simulink model "Linear_Bicycle_Model"  (R2022b)
settings: Solver=ode4  StartTime=0.0  StopTime=20  FixedStep=1e-3  RelTol=1e-3
values from neighbouring files (symbols this model uses):
  Np = 40    [linear_bicycle_script.m]    (also in nonlinear_bicycle_script.m)
  Ts = 0.01    [linear_bicycle_script.m]    (also in nonlinear_bicycle_script.m)
  V_ref = 90 /3.6    (= 25)    [veh_parameters.m]
undefined symbols (not defined in the file or in its folder): data, init, input
settings Model: Creator=nishantc  LastModifiedBy=fiala
settings SolverCC: AlgebraicLoopSolver=TrustRegion
settings DataIOCC: ReturnWorkspaceOutputs=off
settings DebuggingCC: UnconnectedInputMsg=warning  UnconnectedOutputMsg=warning  UnconnectedLineMsg=warning  SFMachineParentedDataDiag=warning  ArithmeticOperatorsInVariantConditions=warning
settings ModelReferenceCC: EnableRefExpFcnMdlSchedulingChecks=on
settings SFSimCC: CustomCodeUndefinedFunction=UseInterfaceOnly
settings RTWCC: DLArmComputeVersion=19.05

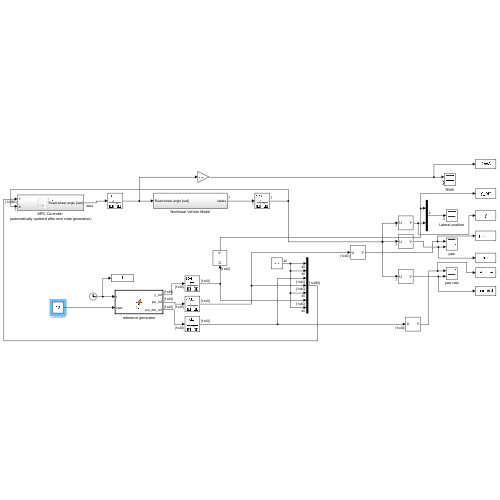
[thumbnail: Simulink's stored preview of the top-level diagram]
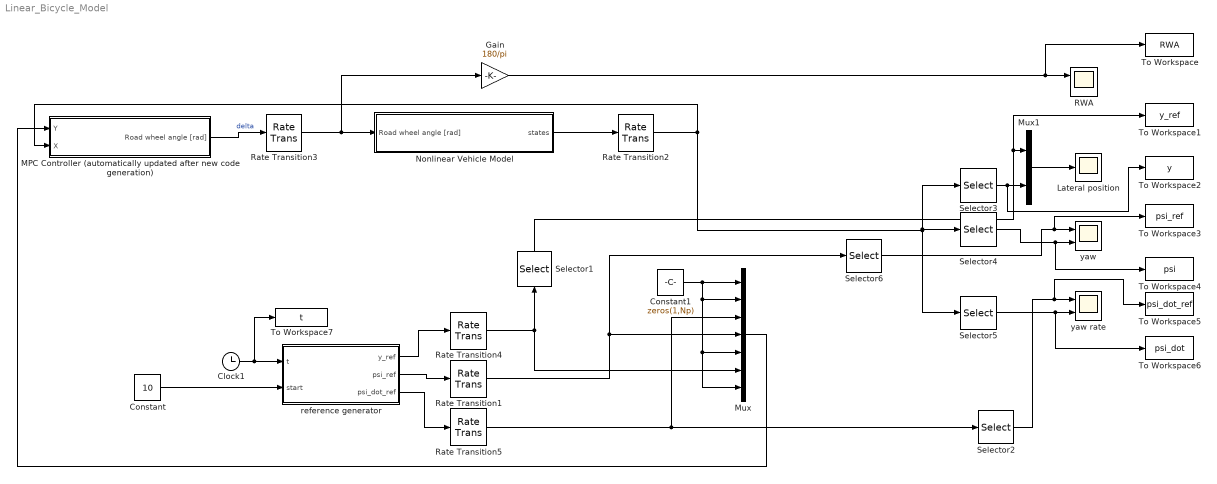
== system Linear_Bicycle_Model ==
  Clock1 : Clock
      settings: Decimation=1000
  Constant : Constant  Value=10
  Constant1 : Constant  Value=zeros(1,Np)
  Gain : Gain  Gain=180/pi
  Lateral position : Scope
  MPC Controller (automatically updated after new code generation) : Subsystem
  Mux : Mux  Inputs=7
  Mux1 : Mux  Inputs=2
  Nonlinear Vehicle Model : Subsystem
  RWA : Scope  NumInputPorts=2
  Rate Transition{1..2,4..5} (4 alike) : RateTransition  OutPortSampleTime=Ts
  Rate Transition3 : RateTransition
  Selector1 : Selector  InputPortWidth=40  IndexOptions=Index vector (dialog)  Indices=1  OutputSizes=1
  Selector2 : Selector  InputPortWidth=40  IndexOptions=Index vector (dialog)  Indices=1  OutputSizes=1
  Selector3 : Selector  InputPortWidth=7  IndexOptions=Index vector (dialog)  Indices=6  OutputSizes=1
  Selector4 : Selector  InputPortWidth=7  IndexOptions=Index vector (dialog)  Indices=4  OutputSizes=1
  Selector5 : Selector  InputPortWidth=7  IndexOptions=Index vector (dialog)  Indices=3  OutputSizes=1
  Selector6 : Selector  InputPortWidth=40  IndexOptions=Index vector (dialog)  Indices=1  OutputSizes=1
  To Workspace : ToWorkspace  VariableName=RWA  SampleTime=-1
  To Workspace1 : ToWorkspace  VariableName=y_ref  SampleTime=-1
  To Workspace2 : ToWorkspace  VariableName=y  SampleTime=-1
  To Workspace3 : ToWorkspace  VariableName=psi_ref  SampleTime=-1
  To Workspace4 : ToWorkspace  VariableName=psi  SampleTime=-1
  To Workspace5 : ToWorkspace  VariableName=psi_dot_ref  SampleTime=-1
  To Workspace6 : ToWorkspace  VariableName=psi_dot  SampleTime=-1
  To Workspace7 : ToWorkspace  VariableName=t  SampleTime=-1
  reference generator : MATLAB Function  TreatAsAtomicUnit=on
  yaw : Scope  NumInputPorts=2
  yaw rate : Scope  NumInputPorts=2
  wires:
  MPC Controller (automatically updated after new code generation)/1(Road wheel angle [rad]) -> Rate Transition3/1  "delta"
  Mux1/1 -> Lateral position/1
  Nonlinear Vehicle Model/1(states) -> Rate Transition2/1
  Selector3/1 -> To Workspace2/1, Mux1/2
  Rate Transition2/1 -> MPC Controller (automatically updated after new code generation)/2(X), Selector3/1, Selector4/1, Selector5/1
  Rate Transition3/1 -> Nonlinear Vehicle Model/1(Road wheel angle [rad]), Gain/1
  Gain/1 -> To Workspace/1, RWA/1
  Mux/1 -> MPC Controller (automatically updated after new code generation)/1(Y)
  Clock1/1 -> To Workspace7/1, reference generator/1(t)
  Constant/1 -> reference generator/2(start)
  reference generator/1(y_ref) -> Rate Transition4/1
  reference generator/2(psi_ref) -> Rate Transition1/1
  reference generator/3(psi_dot_ref) -> Rate Transition5/1
  Selector4/1 -> To Workspace4/1, yaw/2
  Selector5/1 -> To Workspace6/1, yaw rate/2
  Rate Transition1/1 -> Mux/4, Selector6/1
  Rate Transition4/1 -> Selector1/1, Mux/6
  Rate Transition5/1 -> Mux/3, Selector2/1
  Selector1/1 -> To Workspace1/1, Mux1/1
  Selector2/1 -> To Workspace5/1, yaw rate/1
  Selector6/1 -> To Workspace3/1, yaw/1
  Constant1/1 -> Mux/7, Mux/5, Mux/2, Mux/1

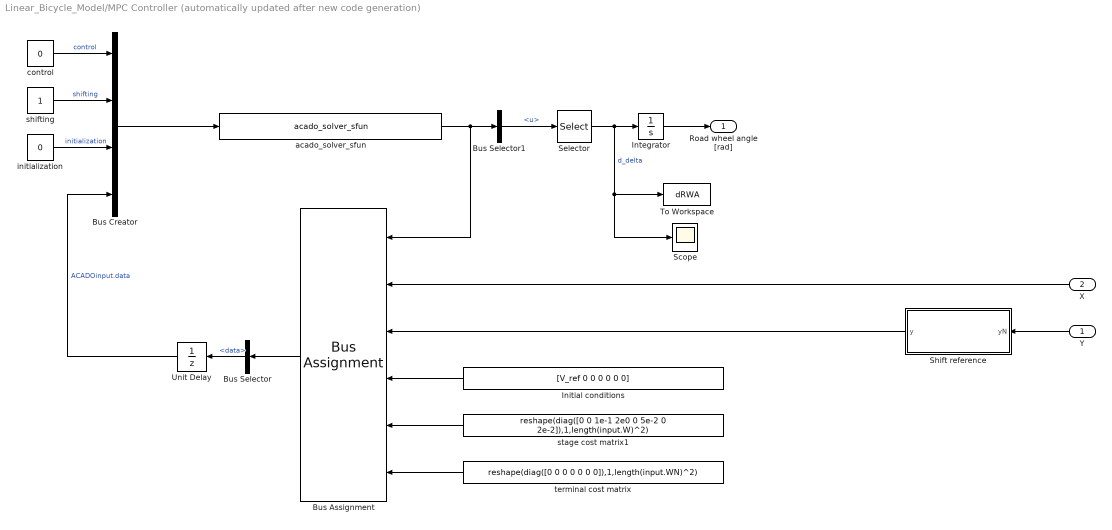
== system Linear_Bicycle_Model/MPC Controller (automatically updated after new code generation) ==
  Y : Inport
  X : Inport  Port=2
  Bus Assignment : BusAssignment  AssignedSignals=data.x0,data.y,data.yN,data.W,data.WN
  Bus Creator : BusCreator  Inputs=4  OutDataTypeStr=Bus: ACADOinput
  Bus Selector : BusSelector  OutputSignals=data
  Bus Selector1 : BusSelector  OutputSignals=data.u
  Initial conditions : Constant  Value=[V_ref 0 0 0 0 0 0]
  Integrator : Integrator
  Scope : Scope
  Selector : Selector  InputPortWidth=Np  IndexOptions=Starting index (dialog)  Indices=[1]  OutputSizes=1
  Shift reference : MATLAB Function  TreatAsAtomicUnit=on
  To Workspace : ToWorkspace  VariableName=dRWA  SampleTime=-1
  Unit Delay : UnitDelay  InitialCondition=init  SampleTime=Ts  HasFrameUpgradeWarning=on
  acado_solver_sfun : S-Function  FunctionName=acado_solver_sfun  SFunctionDeploymentMode=off  EnableBusSupport=off  mask(Legacy Function){SFunctionSpec=acado_step(ACADOinput u1[1], ACADOoutput y1[1]), ShowSpec=on}
      mask prompts: ShowSpec "Display function specification"
      mask help:
      | This block allows you to call the legacy functions specified by the following Legacy Code Tool definition:
      | def.SFunctionName = 'acado_solver_sfun';
      | def.OutputFcnSpec = 'acado_step(ACADOinput u1[1], ACADOoutput y1[1])';
      | def.StartFcnSpec = 'acado_initialize( void )';
      | def.TerminateFcnSpec = 'acado_cleanup( void )';
      | def.HeaderFiles = {'acado_common.h', 'acado_solver_sfunction.h'};
      | def.SourceFiles = {'acado_solver.c', 'acado_integrator.c', 'acado_auxiliary_functions.c', 'acado_solver_sfunction.c', 'acado_qpoases3_interface.c', 'qpoases3\src\Bounds.c', 'qpoases3\src\Constraints.c', 'qpoases3\src\Indexlist.c', 'qpoases3\src\Matrices.c', 'qpoases3\src\MessageHandling.c', 'qpoases3\src\Options.c', 'qpoases3\src\Flipper.c', 'qpoases3\src\QProblem.c', 'qpoases3\src\QProblemB.c', 'qpoases3\src\Utils.c'};
      mask Help: <p>This block was generated automatically by the Legacy Code Tool. For detailed help on this tool, call<a href="matlab:legacy_code('help')"> legacy_code('help')</a>.</p>
      mask Callback ShowSpec:
      | if strcmp(get_param(gcbh, 'ShowSpec'), 'on')
      |   set_param(gcbh, 'MaskDisplay', sprintf('fprintf(''%s'');', get_param(gcbh, 'SFunctionSpec')));
      | else
      |   set_param(gcbh, 'MaskDisplay', sprintf('fprintf(''%s'');', get_param(gcbh, 'FunctionName')));
      | end
      mask Display: fprintf('acado_step(ACADOinput u1[1], ACADOoutput y1[1])');
  control : Constant  Value=0  OutDataTypeStr=int32
  initialization : Constant  Value=0  OutDataTypeStr=int32
  shifting : Constant  OutDataTypeStr=int32
  stage cost matrix1 : Constant  Value=reshape(diag([0 0 1e-1 2e0 0 5e-2 0 2e-2]),1,length(input.W)^2)  VectorParams1D=off
  terminal cost matrix : Constant  Value=reshape(diag([0 0 0 0 0 0 0]),1,length(input.WN)^2)
  Road wheel angle [rad] : Outport
  wires:
  control/1 -> Bus Creator/1  "control"
  Bus Selector1/1 -> Selector/1  "<u>"
  initialization/1 -> Bus Creator/3  "initialization"
  acado_solver_sfun/1 -> Bus Selector1/1, Bus Assignment/1
  shifting/1 -> Bus Creator/2  "shifting"
  X/1 -> Bus Assignment/2
  Bus Assignment/1 -> Bus Selector/1
  terminal cost matrix/1 -> Bus Assignment/6
  Initial conditions/1 -> Bus Assignment/4
  Shift reference/1(y) -> Bus Assignment/3
  stage cost matrix1/1 -> Bus Assignment/5
  Bus Selector/1 -> Unit Delay/1  "<data>"
  Unit Delay/1 -> Bus Creator/4  "ACADOinput.data"
  Bus Creator/1 -> acado_solver_sfun/1
  Y/1 -> Shift reference/1(yN)
  Selector/1 -> Scope/1, To Workspace/1, Integrator/1  "d_delta"
  Integrator/1 -> Road wheel angle [rad]/1

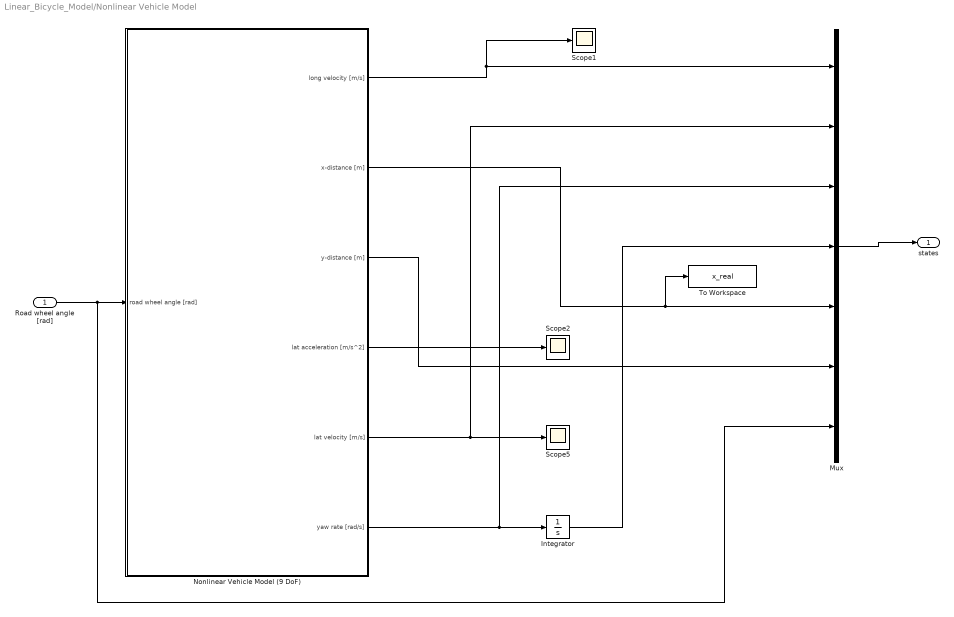
== system Linear_Bicycle_Model/Nonlinear Vehicle Model ==
  Road wheel angle [rad] : Inport
  Integrator : Integrator
  Mux : Mux  Inputs=7
  Nonlinear Vehicle Model (9 DoF) : Subsystem
      mask help: Simulink:masks:GenSFuncDesc_MD
      mask Help: eval('feval(''rtwprivate'',''rtwhelpview'',''rtw_sfcn_block'')');
  Scope1 : Scope
  Scope2 : Scope
  Scope5 : Scope
  To Workspace : ToWorkspace  VariableName=x_real  SampleTime=-1
  states : Outport  VectorParamsAs1DForOutWhenUnconnected=off
  wires:
  Nonlinear Vehicle Model (9 DoF)/4(lat acceleration [m/s^2]) -> Scope2/1
  Nonlinear Vehicle Model (9 DoF)/5(lat velocity [m/s]) -> Mux/2, Scope5/1
  Nonlinear Vehicle Model (9 DoF)/6(yaw rate [rad/s]) -> Mux/3, Integrator/1
  Mux/1 -> states/1
  Nonlinear Vehicle Model (9 DoF)/1(long velocity [m/s]) -> Mux/1, Scope1/1
  Integrator/1 -> Mux/4
  Nonlinear Vehicle Model (9 DoF)/2(x-distance [m]) -> To Workspace/1, Mux/5
  Nonlinear Vehicle Model (9 DoF)/3(y-distance [m]) -> Mux/6
  Road wheel angle [rad]/1 -> Mux/7, Nonlinear Vehicle Model (9 DoF)/1(road wheel angle [rad])

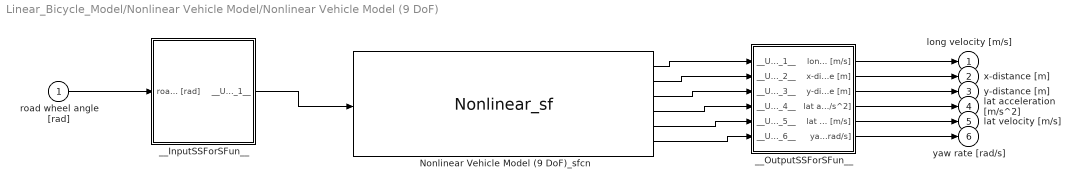
== system Linear_Bicycle_Model/Nonlinear Vehicle Model/Nonlinear Vehicle Model (9 DoF) ==
  road wheel angle [rad] : Inport
  Nonlinear Vehicle Model (9 DoF)_sfcn : S-Function  FunctionName=Nonlinear_sf  SFunctionModules=""  SFunctionDeploymentMode=off  EnableBusSupport=off  mask{rtw_sf_name=Nonlinear_sf, showVar=off}
      mask prompts: rtw_sf_name "Simulink:masks:GenSFuncName_MP"; showVar "Simulink:masks:GenSFuncShowModuleList_MP"
      mask help: Simulink:masks:GenSFuncDesc_MD
      mask init:
      | displist = '';
      | if ~strcmp(get_param(gcb, 'FunctionName'), rtw_sf_name);
      |   set_param(gcb, 'FunctionName', rtw_sf_name);
      | end
      | % Check if we are generating code
      | rtw_mode = false;
      | if strcmpi(get_param(bdroot(gcb),'SimulationStatus'),'Initializing')
      | 	rtw_mode = strcmpi(get_param(bdroot(gcb),'BuildingRTWCode'),'on') && ...
      | 		~strcmpi(get_param(bdroot(gcb),'TargetStyle'),'SimulationTarget');
      | end
      | if showVar || rtw_mode
      | 	if exist('rtwsfunc') == 2 | exist('rtwsfunc') == 6
      | 		tmplist = rtwsfunc(rtw_sf_name,gcb);
      | 		tmplist = DAStudio.message('Simulink:masks:GenSFuncListOfModules_IC', tmplist);
      | 	elseif showVar
      | 		tmplist1 = DAStudio.message('Simulink:masks:GenSFuncListOfModules_IC', '');
      |         tmplist2 = DAStudio.message('Simulink:masks:GenSFuncNotLicensed_IC');
      |         tmplist = [tmplist1 tmplist2];
      |  	end
      | end
      | if showVar
      |   displist = tmplist;
      | end
      settings: CopyFcn=|
      | if ~strcmp(get_param(gcb,'Linkstatus'),'none') && ...
      | ~strcmp(get_param(gcb,'Linkstatus'),'implicit')
      |   set_param(gcb,'LinkStatus','none');
      | end
      mask Help: eval('feval(''rtwprivate'',''rtwhelpview'',''rtw_sfcn_block'')');
      mask Display:
      | port_label('input',1,'road wheel angle [rad]');
      | port_label('output',1,'long velocity [m/s]');
      | port_label('output',2,'x-distance [m]');
      | port_label('output',3,'y-distance [m]');
      | port_label('output',4,'lat acceleration [m/s^2]');
      | port_label('output',5,'lat velocity [m/s]');
      | port_label('output',6,'yaw rate [rad/s]');
  __InputSSForSFun__ : Subsystem
  __OutputSSForSFun__ : Subsystem
  long velocity [m/s] : Outport  VectorParamsAs1DForOutWhenUnconnected=off
  x-distance [m] : Outport  Port=2  VectorParamsAs1DForOutWhenUnconnected=off
  y-distance [m] : Outport  Port=3  VectorParamsAs1DForOutWhenUnconnected=off
  lat acceleration [m/s^2] : Outport  Port=4  VectorParamsAs1DForOutWhenUnconnected=off
  lat velocity [m/s] : Outport  Port=5  VectorParamsAs1DForOutWhenUnconnected=off
  yaw rate [rad/s] : Outport  Port=6  VectorParamsAs1DForOutWhenUnconnected=off
  wires:
  road wheel angle [rad]/1 -> __InputSSForSFun__/1(road wheel angle [rad])
  __InputSSForSFun__/1(__UniqueOutportName__1__) -> Nonlinear Vehicle Model (9 DoF)_sfcn/1
  Nonlinear Vehicle Model (9 DoF)_sfcn/1 -> __OutputSSForSFun__/1(__UniqueInportName__1__)
  Nonlinear Vehicle Model (9 DoF)_sfcn/2 -> __OutputSSForSFun__/2(__UniqueInportName__2__)
  Nonlinear Vehicle Model (9 DoF)_sfcn/3 -> __OutputSSForSFun__/3(__UniqueInportName__3__)
  Nonlinear Vehicle Model (9 DoF)_sfcn/4 -> __OutputSSForSFun__/4(__UniqueInportName__4__)
  Nonlinear Vehicle Model (9 DoF)_sfcn/5 -> __OutputSSForSFun__/5(__UniqueInportName__5__)
  Nonlinear Vehicle Model (9 DoF)_sfcn/6 -> __OutputSSForSFun__/6(__UniqueInportName__6__)
  __OutputSSForSFun__/1(long velocity [m/s]) -> long velocity [m/s]/1
  __OutputSSForSFun__/2(x-distance [m]) -> x-distance [m]/1
  __OutputSSForSFun__/3(y-distance [m]) -> y-distance [m]/1
  __OutputSSForSFun__/4(lat acceleration [m/s^2]) -> lat acceleration [m/s^2]/1
  __OutputSSForSFun__/5(lat velocity [m/s]) -> lat velocity [m/s]/1
  __OutputSSForSFun__/6(yaw rate [rad/s]) -> yaw rate [rad/s]/1

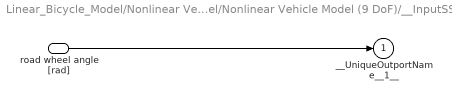
== system Linear_Bicycle_Model/Nonlinear Vehicle Model/Nonlinear Vehicle Model (9 DoF)/__InputSSForSFun__ ==
  road wheel angle [rad] : Inport
  __UniqueOutportName__1__ : Outport
  wires:
  road wheel angle [rad]/1 -> __UniqueOutportName__1__/1

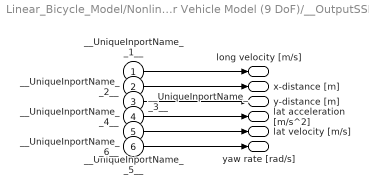
== system Linear_Bicycle_Model/Nonlinear Vehicle Model/Nonlinear Vehicle Model (9 DoF)/__OutputSSForSFun__ ==
  __UniqueInportName__1__ : Inport
  __UniqueInportName__2__ : Inport  Port=2
  __UniqueInportName__3__ : Inport  Port=3
  __UniqueInportName__4__ : Inport  Port=4
  __UniqueInportName__5__ : Inport  Port=5
  __UniqueInportName__6__ : Inport  Port=6
  long velocity [m/s] : Outport  VectorParamsAs1DForOutWhenUnconnected=off
  x-distance [m] : Outport  Port=2  VectorParamsAs1DForOutWhenUnconnected=off
  y-distance [m] : Outport  Port=3  VectorParamsAs1DForOutWhenUnconnected=off
  lat acceleration [m/s^2] : Outport  Port=4  VectorParamsAs1DForOutWhenUnconnected=off
  lat velocity [m/s] : Outport  Port=5  VectorParamsAs1DForOutWhenUnconnected=off
  yaw rate [rad/s] : Outport  Port=6  VectorParamsAs1DForOutWhenUnconnected=off
  wires:
  __UniqueInportName__1__/1 -> long velocity [m/s]/1
  __UniqueInportName__2__/1 -> x-distance [m]/1
  __UniqueInportName__3__/1 -> y-distance [m]/1
  __UniqueInportName__4__/1 -> lat acceleration [m/s^2]/1
  __UniqueInportName__5__/1 -> lat velocity [m/s]/1
  __UniqueInportName__6__/1 -> yaw rate [rad/s]/1

== matlab function Linear_Bicycle_Model/reference generator ==
  data: t input; y_ref output; psi_ref output; psi_dot_ref output; start input; Ts parameter; Np parameter
function [y_ref, psi_ref, psi_dot_ref] = fcn(t, start, Ts, Np)
    y_ref = zeros(1, 40);
    psi_ref = zeros(1, 40);
    psi_dot_ref = zeros(1, 40);
    % Define the parameters
    B = 2.8; % Example value
    x1 = 30; % Example value
    y1 = 0.92; % Example value
    y_tol = 0.3; % Example value
    C1 = log((B/y_tol) - 1);
    C2 = 5; % Example value
    Vx = 90 / 3.6;

    % Calculate k1, k2, k3
    k1 = (B * x1)^2 / 16 - (B * C2)^2 / 16;
    k2 = -B^2 * x1 * C1 / 8 - B * y1 * x1 / 2 + B^2 * x1 / 4;
    k3 = (B * C1)^2 / 16 + y1^2 + B^2 / 4 + B * y1 * C1 /2 - B * y1 - B^2 * C1 / 4 - C2^2;

    % Calculate a and c
    a = (-k2 + sqrt(k2^2 - 4 * k1 * k3)) / (2 * k1);
    c = C1 / a;

    timing = t-start:0.01:t-start+40*0.01-0.01;
    % Define the range of x
    x = Vx * timing;

    % Compute y_ref
    y_ref(timing' < 0) = y_tol;
    y_ref(timing' >= 0) = B ./ (1 + exp(-a * (x(timing>=0) - c)));

    % Compute the first derivative of y_ref with respect to x
%     dydx = gradient(y_ref, x);
    x(timing < 0) = 0;
    dydx = (B*a*exp(a*(c - x)))./(exp(a*(c - x)) + 1).^2;


    % Compute the second derivative of y_ref with respect to x
%     d2ydx2 = gradient(dydx, x);
    d2ydx2 = (2*B*a^2*exp(2*a*(c - x)))./(exp(a*(c - x)) + 1).^3 ...
        - (B*a^2*exp(a*(c - x)))./(exp(a*(c - x)) + 1).^2;

    % Define the expression for kappa_1
    kappa_1 = d2ydx2 ./ (1 + dydx.^2).^(3/2);

    % Compute psi_ref
    psi_ref(1:end) = atan(dydx);
    psi_ref(timing < 0) = 0;

    % Compute psi_dot_ref
    psi_dot_ref(1:end) = kappa_1 * Vx;
    psi_dot_ref(timing < 0) = 0;
end

== matlab function Linear_Bicycle_Model/MPC Controller (automatically updated after new code generation)/Shift reference ==
  data: y output; yN input; Np parameter
function y = shift_reference(yN,Np)

a = reshape(yN, Np, 7)'; % have a column for each timestep
b = [a; zeros(size(a(1, :)))]; % add input
y = reshape(b, 1, Np*8);

% y=repmat([yN;0],Np,1)';
% y = zeros(1, 40*8);

end
